simulink model "wrist_imu_main"  (R2025a)
settings: Solver=FixedStepDiscrete  StartTime=0.0  StopTime=T  FixedStep=Ts  RelTol=1e-3
undefined symbols (not defined in the file): imu
settings Model: Creator=CSY  LastModifiedBy=CSY

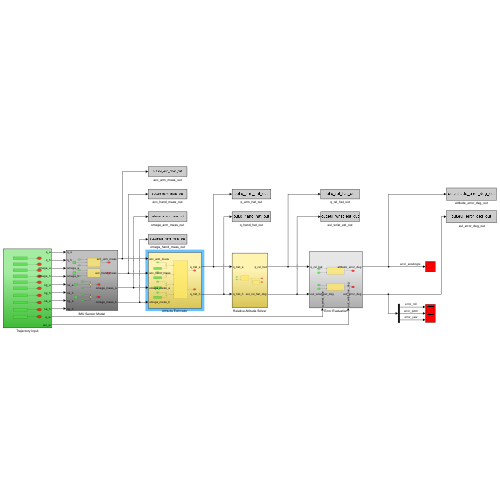
[thumbnail: Simulink's stored preview of the top-level diagram]
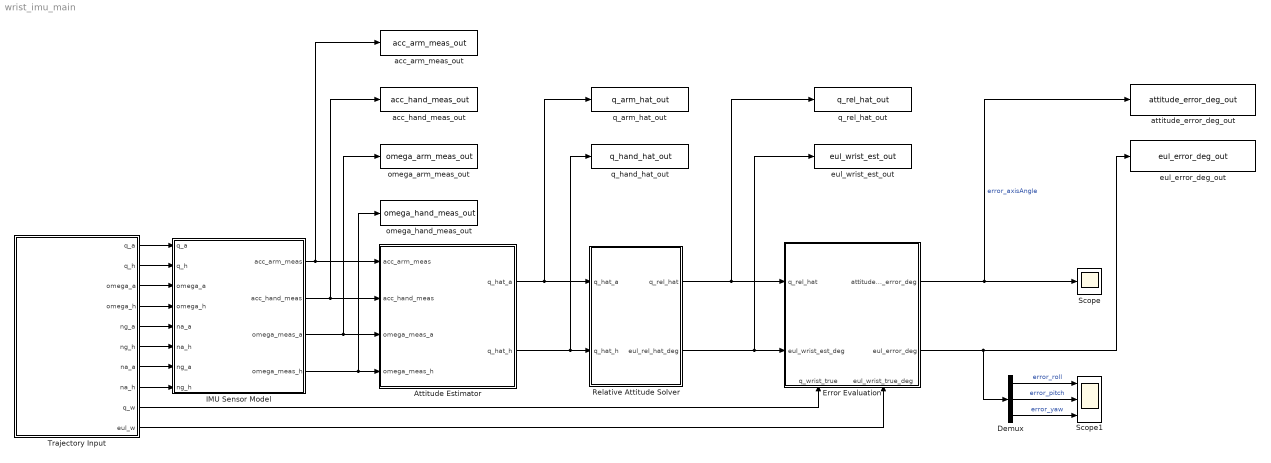
== system wrist_imu_main ==
  " eul_error_deg_out" : ToWorkspace  VariableName=eul_error_deg_out  SaveFormat=Timeseries  SampleTime=-1
  Attitude Estimator : Subsystem
  Demux : Demux  Outputs=3
  Error Evaluation : Subsystem
      settings: PortSchema="{\"entries\":[{\"content\":{\"sides\":[{\"content\":{\"connectorIds\":[\"In1\",\"In2\"]},\"type\":\"ConnectorPlacement.EquallySpacedRectSide\",\"uuid\":\"abe2ae72-a5a0-403c-9e03-1b4f6d4d0d67\"},{\"content\":{\"connectorIds\":[\"Out1\",\"Out2\"],\"side\":\"RIGHT\"},\"type\":\"ConnectorPlacement.EquallySpacedRectSide\",\"uuid\":\"685a4192-adf4-4593-bc2e-0bd30f7cac66\"},{\"content\":{\"side\":\"TOP\"},\"type\":\"ConnectorPlacement.EquallySpacedRectSide\",\"uuid\":\"39d5cefb-5657-4ba3-9dd7-93d12642c754\"},{\"content\":{\"connectorIds\":[\"In3\",\"In4\"],\"side\":\"BOTTOM\"},\"type\":\"ConnectorPlacement.EquallySpacedRectSide\",\"uuid\":\"5c41fd23-46de-49da-8620-9a3bda566928\"}]},\"type\":\"ConnectorPlacement.EquallySpacedConnector\",\"uuid\":\"e8722cc7-0898-4a9c-a259-ee97117e6560\"}],\"packageUris\":[\"http://schema.mathworks.com/mf0/Connector/R2020b\"],\"version\":\"1.0\"}"
  IMU Sensor Model : Subsystem
  Relative Attitude Solver : Subsystem
  Scope : Scope
      settings: ActiveDisplayYMinimum=-0.17689613299070039  ActiveDisplayYMaximum=0.60715026770063385
  Scope1 : Scope  NumInputPorts=3
      settings: ActiveDisplayYMinimum=-51.230869792156561  ActiveDisplayYMaximum=63.683087774127145
  Trajectory Input : Subsystem
  acc_arm_meas_out : ToWorkspace  VariableName=acc_arm_meas_out  SaveFormat=Timeseries  SampleTime=-1
  acc_hand_meas_out : ToWorkspace  VariableName=acc_hand_meas_out  SaveFormat=Timeseries  SampleTime=-1
  attitude_error_deg_out : ToWorkspace  VariableName=attitude_error_deg_out  SaveFormat=Timeseries  SampleTime=-1
  eul_wrist_est_out : ToWorkspace  VariableName=eul_wrist_est_out  SaveFormat=Timeseries  SampleTime=-1
  omega_arm_meas_out : ToWorkspace  VariableName=omega_arm_meas_out  SaveFormat=Timeseries  SampleTime=-1
  omega_hand_meas_out : ToWorkspace  VariableName=omega_hand_meas_out  SaveFormat=Timeseries  SampleTime=-1
  q_arm_hat_out : ToWorkspace  VariableName=q_arm_hat_out  SaveFormat=Timeseries  SampleTime=-1
  q_hand_hat_out : ToWorkspace  VariableName=q_hand_hat_out  SaveFormat=Timeseries  SampleTime=-1
  q_rel_hat_out : ToWorkspace  VariableName=q_rel_hat_out  SaveFormat=Timeseries  SampleTime=-1
  wires:
  Trajectory Input/3(omega_a) -> IMU Sensor Model/3(omega_a)
  Trajectory Input/4(omega_h) -> IMU Sensor Model/4(omega_h)
  IMU Sensor Model/3(omega_meas_a) -> omega_arm_meas_out/1, Attitude Estimator/3(omega_meas_a)
  IMU Sensor Model/4(omega_meas_h) -> omega_hand_meas_out/1, Attitude Estimator/4(omega_meas_h)
  Attitude Estimator/1(q_hat_a) -> Relative Attitude Solver/1(q_hat_a), q_arm_hat_out/1
  Attitude Estimator/2(q_hat_h) -> q_hand_hat_out/1, Relative Attitude Solver/2(q_hat_h)
  Relative Attitude Solver/1(q_rel_hat) -> q_rel_hat_out/1, Error Evaluation/1(q_rel_hat)
  Relative Attitude Solver/2(eul_rel_hat_deg) -> eul_wrist_est_out/1, Error Evaluation/2(eul_wrist_est_deg)
  Trajectory Input/9(q_w) -> Error Evaluation/3(q_wrist_true)
  Trajectory Input/10(eul_w) -> Error Evaluation/4(eul_wrist_true_deg)
  Error Evaluation/1(attitude_error_deg) -> attitude_error_deg_out/1, Scope/1  "error_axisAngle"
  Error Evaluation/2(eul_error_deg) -> Demux/1, " eul_error_deg_out"/1
  Demux/2 -> Scope1/2  "error_pitch"
  Demux/1 -> Scope1/1  "error_roll"
  Demux/3 -> Scope1/3  "error_yaw"
  Trajectory Input/1(q_a) -> IMU Sensor Model/1(q_a)
  Trajectory Input/2(q_h) -> IMU Sensor Model/2(q_h)
  IMU Sensor Model/1(acc_arm_meas) -> acc_arm_meas_out/1, Attitude Estimator/1(acc_arm_meas)
  IMU Sensor Model/2(acc_hand_meas) -> acc_hand_meas_out/1, Attitude Estimator/2(acc_hand_meas)
  Trajectory Input/5(ng_a) -> IMU Sensor Model/5(na_a)
  Trajectory Input/6(ng_h) -> IMU Sensor Model/6(na_h)
  Trajectory Input/7(na_a) -> IMU Sensor Model/7(ng_a)
  Trajectory Input/8(na_h) -> IMU Sensor Model/8(ng_h)

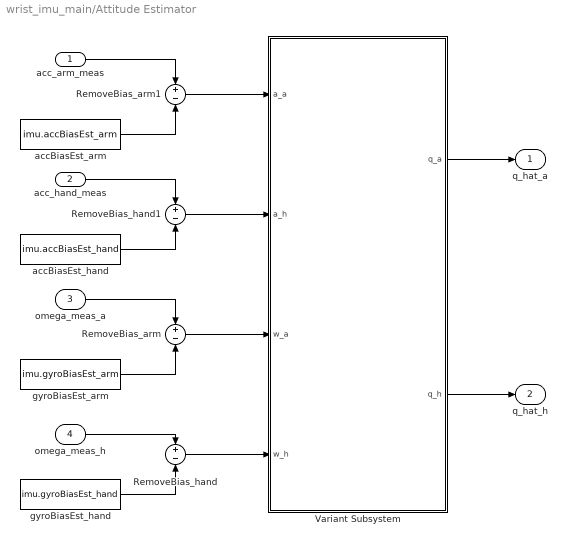
== system wrist_imu_main/Attitude Estimator ==
  acc_arm_meas : Inport
  acc_hand_meas : Inport  Port=2
  omega_meas_a : Inport  Port=3
  omega_meas_h : Inport  Port=4
  RemoveBias_arm : Sum  Inputs=+-
  RemoveBias_arm1 : Sum  Inputs=+-
  RemoveBias_hand : Sum  Inputs=+-
  RemoveBias_hand1 : Sum  Inputs=+-
  Variant Subsystem : Subsystem  Variant=on
  accBiasEst_arm : Constant  Value=imu.accBiasEst_arm
  accBiasEst_hand : Constant  Value=imu.accBiasEst_hand
  gyroBiasEst_arm : Constant  Value=imu.gyroBiasEst_arm
  gyroBiasEst_hand : Constant  Value=imu.gyroBiasEst_hand
  q_hat_a : Outport
  q_hat_h : Outport  Port=2
  wires:
  omega_meas_a/1 -> RemoveBias_arm/1
  gyroBiasEst_arm/1 -> RemoveBias_arm/2
  omega_meas_h/1 -> RemoveBias_hand/1
  gyroBiasEst_hand/1 -> RemoveBias_hand/2
  RemoveBias_arm/1 -> Variant Subsystem/3(w_a)
  Variant Subsystem/1(q_a) -> q_hat_a/1
  RemoveBias_hand/1 -> Variant Subsystem/4(w_h)
  Variant Subsystem/2(q_h) -> q_hat_h/1
  acc_arm_meas/1 -> RemoveBias_arm1/1
  acc_hand_meas/1 -> RemoveBias_hand1/1
  accBiasEst_arm/1 -> RemoveBias_arm1/2
  RemoveBias_arm1/1 -> Variant Subsystem/1(a_a)
  accBiasEst_hand/1 -> RemoveBias_hand1/2
  RemoveBias_hand1/1 -> Variant Subsystem/2(a_h)

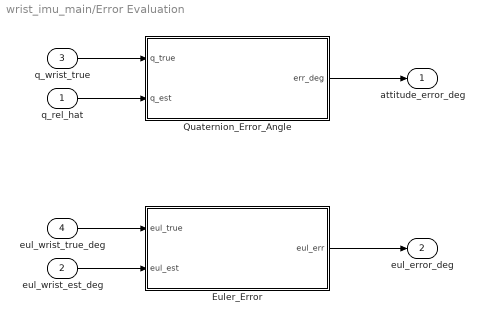
== system wrist_imu_main/Error Evaluation ==
  q_rel_hat : Inport
  eul_wrist_est_deg : Inport  Port=2
  q_wrist_true : Inport  Port=3
  eul_wrist_true_deg : Inport  Port=4
  Euler_Error : MATLAB Function  TreatAsAtomicUnit=on
  Quaternion_Error_Angle : MATLAB Function  TreatAsAtomicUnit=on
  attitude_error_deg : Outport
  eul_error_deg : Outport  Port=2
  wires:
  q_wrist_true/1 -> Quaternion_Error_Angle/1(q_true)
  q_rel_hat/1 -> Quaternion_Error_Angle/2(q_est)
  Quaternion_Error_Angle/1(err_deg) -> attitude_error_deg/1
  eul_wrist_true_deg/1 -> Euler_Error/1(eul_true)
  eul_wrist_est_deg/1 -> Euler_Error/2(eul_est)
  Euler_Error/1(eul_err) -> eul_error_deg/1

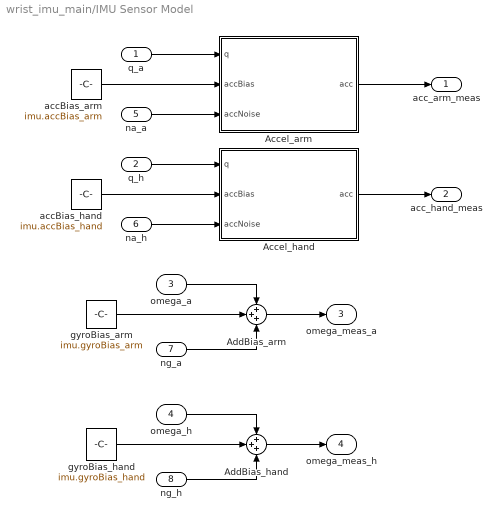
== system wrist_imu_main/IMU Sensor Model ==
  q_a : Inport
  q_h : Inport  Port=2
  omega_a : Inport  Port=3
  omega_h : Inport  Port=4
  na_a : Inport  Port=5
  na_h : Inport  Port=6
  ng_a : Inport  Port=7
  ng_h : Inport  Port=8
  Accel_arm : MATLAB Function  TreatAsAtomicUnit=on
  Accel_hand : MATLAB Function  TreatAsAtomicUnit=on
  AddBias_arm : Sum  Inputs=+++
  AddBias_hand : Sum  Inputs=+++
  accBias_arm : Constant  Value=imu.accBias_arm
  accBias_hand : Constant  Value=imu.accBias_hand
  gyroBias_arm : Constant  Value=imu.gyroBias_arm
  gyroBias_hand : Constant  Value=imu.gyroBias_hand
  acc_arm_meas : Outport
  acc_hand_meas : Outport  Port=2
  omega_meas_a : Outport  Port=3
  omega_meas_h : Outport  Port=4
  wires:
  omega_a/1 -> AddBias_arm/1
  gyroBias_arm/1 -> AddBias_arm/2
  AddBias_arm/1 -> omega_meas_a/1
  omega_h/1 -> AddBias_hand/1
  gyroBias_hand/1 -> AddBias_hand/2
  AddBias_hand/1 -> omega_meas_h/1
  q_h/1 -> Accel_hand/1(q)
  q_a/1 -> Accel_arm/1(q)
  Accel_arm/1(acc) -> acc_arm_meas/1
  Accel_hand/1(acc) -> acc_hand_meas/1
  accBias_hand/1 -> Accel_hand/2(accBias)
  accBias_arm/1 -> Accel_arm/2(accBias)
  na_h/1 -> Accel_hand/3(accNoise)
  na_a/1 -> Accel_arm/3(accNoise)
  ng_h/1 -> AddBias_hand/3
  ng_a/1 -> AddBias_arm/3

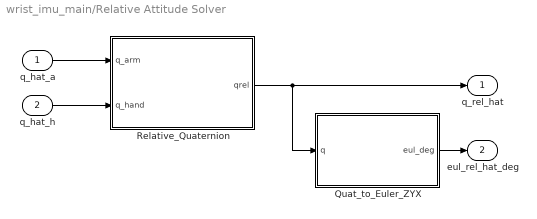
== system wrist_imu_main/Relative Attitude Solver ==
  q_hat_a : Inport
  q_hat_h : Inport  Port=2
  Quat_to_Euler_ZYX : MATLAB Function  TreatAsAtomicUnit=on
  Relative_Quaternion : MATLAB Function  TreatAsAtomicUnit=on
  q_rel_hat : Outport
  eul_rel_hat_deg : Outport  Port=2
  wires:
  q_hat_a/1 -> Relative_Quaternion/1(q_arm)
  q_hat_h/1 -> Relative_Quaternion/2(q_hand)
  Relative_Quaternion/1(qrel) -> Quat_to_Euler_ZYX/1(q), q_rel_hat/1
  Quat_to_Euler_ZYX/1(eul_deg) -> eul_rel_hat_deg/1

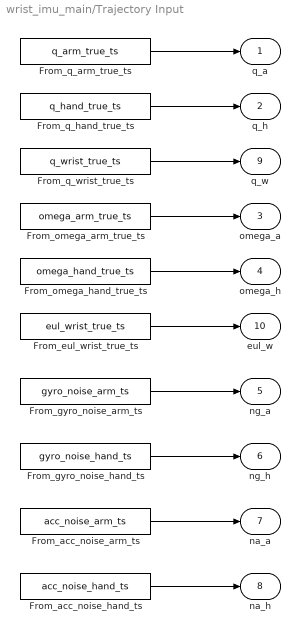
== system wrist_imu_main/Trajectory Input ==
  From_acc_noise_arm_ts : FromWorkspace  VariableName=acc_noise_arm_ts
  From_acc_noise_hand_ts : FromWorkspace  VariableName=acc_noise_hand_ts
  From_eul_wrist_true_ts : FromWorkspace  VariableName=eul_wrist_true_ts
  From_gyro_noise_arm_ts : FromWorkspace  VariableName=gyro_noise_arm_ts
  From_gyro_noise_hand_ts : FromWorkspace  VariableName=gyro_noise_hand_ts
  From_omega_arm_true_ts : FromWorkspace  VariableName=omega_arm_true_ts
  From_omega_hand_true_ts : FromWorkspace  VariableName=omega_hand_true_ts
  From_q_arm_true_ts : FromWorkspace  VariableName=q_arm_true_ts
  From_q_hand_true_ts : FromWorkspace  VariableName=q_hand_true_ts
  From_q_wrist_true_ts : FromWorkspace  VariableName=q_wrist_true_ts
  q_a : Outport
  q_h : Outport  Port=2
  omega_a : Outport  Port=3
  omega_h : Outport  Port=4
  ng_a : Outport  Port=5
  ng_h : Outport  Port=6
  na_a : Outport  Port=7
  na_h : Outport  Port=8
  q_w : Outport  Port=9
  eul_w : Outport  Port=10
  wires:
  From_q_arm_true_ts/1 -> q_a/1
  From_q_hand_true_ts/1 -> q_h/1
  From_q_wrist_true_ts/1 -> q_w/1
  From_omega_arm_true_ts/1 -> omega_a/1
  From_omega_hand_true_ts/1 -> omega_h/1
  From_eul_wrist_true_ts/1 -> eul_w/1
  From_gyro_noise_arm_ts/1 -> ng_a/1
  From_gyro_noise_hand_ts/1 -> ng_h/1
  From_acc_noise_arm_ts/1 -> na_a/1
  From_acc_noise_hand_ts/1 -> na_h/1

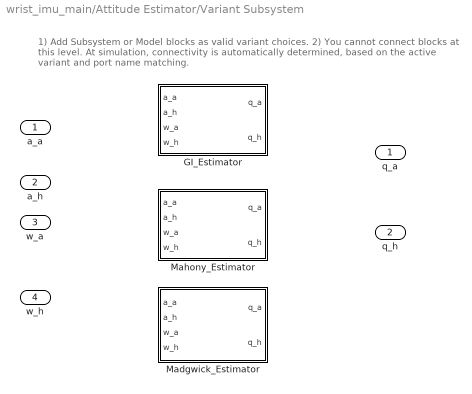
== system wrist_imu_main/Attitude Estimator/Variant Subsystem ==
  note: 1) Add Subsystem or Model blocks as valid variant choices.
      | 2) You cannot connect blocks at this level. At simulation, connectivity is automatically
      | determined, based on the active variant and port name matching.
  a_a : Inport
  a_h : Inport  Port=2
  w_a : Inport  Port=3
  w_h : Inport  Port=4
  GI_Estimator : Subsystem  VariantControl=ESTIMATOR == 1
  Madgwick_Estimator : Subsystem  VariantControl=ESTIMATOR == 3
  Mahony_Estimator : Subsystem  VariantControl=ESTIMATOR == 2
  q_a : Outport
  q_h : Outport  Port=2

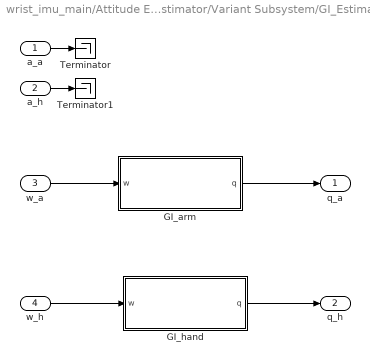
== system wrist_imu_main/Attitude Estimator/Variant Subsystem/GI_Estimator ==
  a_a : Inport
  a_h : Inport  Port=2
  w_a : Inport  Port=3
  w_h : Inport  Port=4
  GI_arm : MATLAB Function  TreatAsAtomicUnit=on
  GI_hand : MATLAB Function  TreatAsAtomicUnit=on
  Terminator : Terminator
  Terminator1 : Terminator
  q_a : Outport
  q_h : Outport  Port=2
  wires:
  w_h/1 -> GI_hand/1(w)
  GI_arm/1(q) -> q_a/1
  GI_hand/1(q) -> q_h/1
  w_a/1 -> GI_arm/1(w)
  a_a/1 -> Terminator/1
  a_h/1 -> Terminator1/1

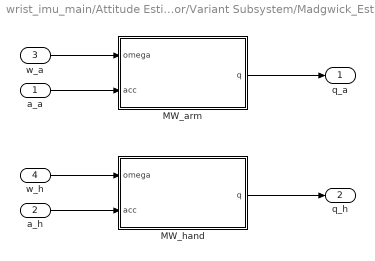
== system wrist_imu_main/Attitude Estimator/Variant Subsystem/Madgwick_Estimator ==
  a_a : Inport
  a_h : Inport  Port=2
  w_a : Inport  Port=3
  w_h : Inport  Port=4
  MW_arm : MATLAB Function  TreatAsAtomicUnit=on
  MW_hand : MATLAB Function  TreatAsAtomicUnit=on
  q_a : Outport
  q_h : Outport  Port=2
  wires:
  w_h/1 -> MW_hand/1(omega)
  w_a/1 -> MW_arm/1(omega)
  MW_hand/1(q) -> q_h/1
  MW_arm/1(q) -> q_a/1
  a_a/1 -> MW_arm/2(acc)
  a_h/1 -> MW_hand/2(acc)

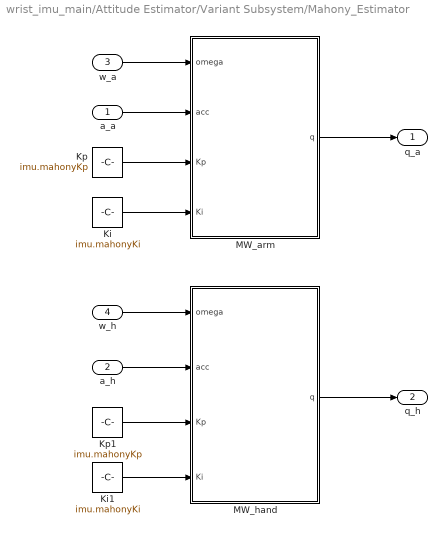
== system wrist_imu_main/Attitude Estimator/Variant Subsystem/Mahony_Estimator ==
  a_a : Inport
  a_h : Inport  Port=2
  w_a : Inport  Port=3
  w_h : Inport  Port=4
  Ki : Constant  Value=imu.mahonyKi
  Ki1 : Constant  Value=imu.mahonyKi
  Kp : Constant  Value=imu.mahonyKp
  Kp1 : Constant  Value=imu.mahonyKp
  MW_arm : MATLAB Function  TreatAsAtomicUnit=on
  MW_hand : MATLAB Function  TreatAsAtomicUnit=on
  q_a : Outport
  q_h : Outport  Port=2
  wires:
  w_a/1 -> MW_arm/1(omega)
  w_h/1 -> MW_hand/1(omega)
  MW_arm/1(q) -> q_a/1
  a_h/1 -> MW_hand/2(acc)
  MW_hand/1(q) -> q_h/1
  a_a/1 -> MW_arm/2(acc)
  Kp/1 -> MW_arm/3(Kp)
  Ki/1 -> MW_arm/4(Ki)
  Kp1/1 -> MW_hand/3(Kp)
  Ki1/1 -> MW_hand/4(Ki)

== matlab function wrist_imu_main/IMU Sensor Model/Accel_hand ==
  data: q input; acc output; accBias input; accNoise input
function acc = Accel_Model(q, accBias, accNoise)
%#codegen
% q: [w x y z], body -> world
% acc: body frame accelerometer output, m/s^2

q = q(:);
q = q / norm(q);

w = q(1);
x = q(2);
y = q(3);
z = q(4);

R = zeros(3,3);

R(1,1) = 1 - 2*(y^2 + z^2);
R(1,2) = 2*(x*y - w*z);
R(1,3) = 2*(x*z + w*y);

R(2,1) = 2*(x*y + w*z);
R(2,2) = 1 - 2*(x^2 + z^2);
R(2,3) = 2*(y*z - w*x);

R(3,1) = 2*(x*z - w*y);
R(3,2) = 2*(y*z + w*x);
R(3,3) = 1 - 2*(x^2 + y^2);

g_W = [0; 0; 9.81];

acc = R' * g_W + accBias(:) + accNoise(:);
end

== matlab function wrist_imu_main/IMU Sensor Model/Accel_arm ==
  data: q input; acc output; accBias input; accNoise input
function acc = Accel_Model(q, accBias, accNoise)
%#codegen
% q: [w x y z], body -> world
% acc: body frame accelerometer output, m/s^2

q = q(:);
q = q / norm(q);

w = q(1);
x = q(2);
y = q(3);
z = q(4);

R = zeros(3,3);

R(1,1) = 1 - 2*(y^2 + z^2);
R(1,2) = 2*(x*y - w*z);
R(1,3) = 2*(x*z + w*y);

R(2,1) = 2*(x*y + w*z);
R(2,2) = 1 - 2*(x^2 + z^2);
R(2,3) = 2*(y*z - w*x);

R(3,1) = 2*(x*z - w*y);
R(3,2) = 2*(y*z + w*x);
R(3,3) = 1 - 2*(x^2 + y^2);

g_W = [0; 0; 9.81];

acc = R' * g_W + accBias(:) + accNoise(:);
end

== matlab function wrist_imu_main/Relative Attitude Solver/Relative_Quaternion ==
  data: q_arm input; qrel output; q_hand input
function qrel = Relative_Quaternion(q_arm, q_hand)
%#codegen
% qrel = q_arm^{-1} ⊗ q_hand
% 四元数格式：[w x y z]，标量在前

q_arm = q_arm(:);
q_hand = q_hand(:);

q_arm = q_arm / norm(q_arm);
q_hand = q_hand / norm(q_hand);

% q_arm 的逆：单位四元数的逆等于共轭
q1 = zeros(4,1);
q1(1) = q_arm(1);
q1(2:4) = -q_arm(2:4);

q2 = q_hand;

% qrel = q1 ⊗ q2
s1 = q1(1);
v1 = q1(2:4);
s2 = q2(1);
v2 = q2(2:4);

qrel = zeros(4,1);
qrel(1) = s1*s2 - dot(v1,v2);
qrel(2:4) = s1*v2 + s2*v1 + cross(v1,v2);

qrel = qrel / norm(qrel);

% 统一符号，避免 q 和 -q 跳变
if qrel(1) < 0
    qrel = -qrel;
end
end

== matlab function wrist_imu_main/Relative Attitude Solver/Quat_to_Euler_ZYX ==
  data: q input; eul_deg output
function eul_deg = Quat_to_Euler_ZYX(q)
%#codegen
% 输入 q: [w x y z]
% 输出 eul_deg = [roll pitch yaw]，单位 deg
% 欧拉角顺序：ZYX，即 R = Rz(yaw) * Ry(pitch) * Rx(roll)

q = q(:);
q = q / norm(q);

w = q(1);
x = q(2);
y = q(3);
z = q(4);

R11 = 1 - 2*(y^2 + z^2);
R21 = 2*(x*y + w*z);
R31 = 2*(x*z - w*y);
R32 = 2*(y*z + w*x);
R33 = 1 - 2*(x^2 + y^2);

% 防止数值误差导致 asin 输入略超 [-1,1]
v = -R31;
if v > 1
    v = 1;
elseif v < -1
    v = -1;
end

pitch = asin(v);
roll  = atan2(R32, R33);
yaw   = atan2(R21, R11);

eul_deg = [roll; pitch; yaw] * 180/pi;

== matlab function wrist_imu_main/Error Evaluation/Quaternion_Error_Angle ==
  data: q_true input; err_deg output; q_est input
function err_deg = Quaternion_Error_Angle(q_true, q_est)
%#codegen
% 计算 q_true 和 q_est 之间的姿态误差角，单位 deg

q_true = q_true(:);
q_est = q_est(:);

q_true = q_true / norm(q_true);
q_est = q_est / norm(q_est);

% qerr = q_true^{-1} ⊗ q_est
q1 = zeros(4,1);
q1(1) = q_true(1);
q1(2:4) = -q_true(2:4);

q2 = q_est;

s1 = q1(1);
v1 = q1(2:4);
s2 = q2(1);
v2 = q2(2:4);

qerr = zeros(4,1);
qerr(1) = s1*s2 - dot(v1,v2);
qerr(2:4) = s1*v2 + s2*v1 + cross(v1,v2);
qerr = qerr / norm(qerr);

% q 和 -q 表示同一姿态，所以取 abs
c = abs(qerr(1));
if c > 1
    c = 1;
end

err_deg = 2 * acos(c) * 180/pi;
end

== matlab function wrist_imu_main/Error Evaluation/Euler_Error ==
  data: eul_true input; eul_err output; eul_est input
function eul_err = Euler_Error(eul_true, eul_est)
%#codegen
% 输入单位 deg，输出 eul_est - eul_true

eul_true = eul_true(:);
eul_est = eul_est(:);

eul_err = zeros(3,1);
eul_err = eul_est - eul_true;

% 简单处理角度跨越 ±180 的情况
for i = 1:3
    if eul_err(i) > 180
        eul_err(i) = eul_err(i) - 360;
    elseif eul_err(i) < -180
        eul_err(i) = eul_err(i) + 360;
    end
end
end

== matlab function wrist_imu_main/Attitude Estimator/Variant Subsystem/GI_Estimator/GI_arm ==
  data: w input; q output
function q = GI_Quat_Integrator(w)
%#codegen

% 输入 w: 3维角速度，单位 rad/s
% 输出 q: 4x1 四元数 [w x y z]

persistent qk
Ts = 0.01;

if isempty(qk)
    qk = zeros(4,1);
    qk(1) = 1;
end

w = w(:);
theta = norm(w) * Ts;

if theta < 1e-12
    dq = zeros(4,1);
    dq(1) = 1;
    dq(2:4) = 0.5 * w * Ts;
else
    axis = w / norm(w);
    dq = zeros(4,1);
    dq(1) = cos(theta/2);
    dq(2:4) = axis * sin(theta/2);
end

% qk = qk ⊗ dq
s1 = qk(1);
v1 = qk(2:4);
s2 = dq(1);
v2 = dq(2:4);

qnew = zeros(4,1);
qnew(1) = s1*s2 - dot(v1,v2);
qnew(2:4) = s1*v2 + s2*v1 + cross(v1,v2);

qk = qnew / norm(qnew);
q = qk;
end

== matlab function wrist_imu_main/Attitude Estimator/Variant Subsystem/GI_Estimator/GI_hand ==
  data: w input; q output
function q = GI_Quat_Integrator(w)
%#codegen

% 输入 w: 3维角速度，单位 rad/s
% 输出 q: 4x1 四元数 [w x y z]

persistent qk
Ts = 0.01;

if isempty(qk)
    qk = zeros(4,1);
    qk(1) = 1;
end

w = w(:);
theta = norm(w) * Ts;

if theta < 1e-12
    dq = zeros(4,1);
    dq(1) = 1;
    dq(2:4) = 0.5 * w * Ts;
else
    axis = w / norm(w);
    dq = zeros(4,1);
    dq(1) = cos(theta/2);
    dq(2:4) = axis * sin(theta/2);
end

% qk = qk ⊗ dq
s1 = qk(1);
v1 = qk(2:4);
s2 = dq(1);
v2 = dq(2:4);

qnew = zeros(4,1);
qnew(1) = s1*s2 - dot(v1,v2);
qnew(2:4) = s1*v2 + s2*v1 + cross(v1,v2);

qk = qnew / norm(qnew);
q = qk;
end

== matlab function wrist_imu_main/Attitude Estimator/Variant Subsystem/Madgwick_Estimator/MW_arm ==
  data: omega input; q output; acc input
function q = Mahony_IMU(omega, acc)
%#codegen
% omega: 3x1 rad/s
% acc:   3x1 m/s^2
% q:     4x1 quaternion [w x y z]
%
% q 表示 body -> world 的姿态

persistent qk intErr

Ts = 0.01;
Kp = 2.0;
Ki = 0.05;

if isempty(qk)
    qk = [1;0;0;0];
    intErr = [0;0;0];
end

omega = omega(:);
acc = acc(:);

% 加速度归一化，只保留方向
accNorm = norm(acc);
if accNorm > 1e-8
    a = acc / accNorm;
else
    a = [0;0;1];
end

% 当前四元数
qk = qk / norm(qk);

w = qk(1);
x = qk(2);
y = qk(3);
z = qk(4);

% R: body -> world
R = zeros(3,3);
R(1,1) = 1 - 2*(y^2 + z^2);
R(1,2) = 2*(x*y - w*z);
R(1,3) = 2*(x*z + w*y);

R(2,1) = 2*(x*y + w*z);
R(2,2) = 1 - 2*(x^2 + z^2);
R(2,3) = 2*(y*z - w*x);

R(3,1) = 2*(x*z - w*y);
R(3,2) = 2*(y*z + w*x);
R(3,3) = 1 - 2*(x^2 + y^2);

% 预测的重力方向在 body 坐标系下的表达
g_world = [0;0;1];
g_hat_body = R' * g_world;

% 姿态误差：测得重力方向 vs 预测重力方向
e = cross(a, g_hat_body);

% 积分项，用于补偿陀螺零偏
intErr = intErr + e * Ts;

% 修正角速度
omega_corr = omega + Kp * e + Ki * intErr;

% 四元数积分
theta = norm(omega_corr) * Ts;

if theta < 1e-12
    dq = [1; 0.5 * omega_corr * Ts];
else
    axis = omega_corr / norm(omega_corr);
    dq = [cos(theta/2); axis * sin(theta/2)];
end

% qk = qk ⊗ dq
s1 = qk(1); v1 = qk(2:4);
s2 = dq(1); v2 = dq(2:4);

qnew = zeros(4,1);
qnew(1) = s1*s2 - dot(v1,v2);
qnew(2:4) = s1*v2 + s2*v1 + cross(v1,v2);

qk = qnew / norm(qnew);
q = qk;
end

== matlab function wrist_imu_main/Attitude Estimator/Variant Subsystem/Madgwick_Estimator/MW_hand ==
  data: omega input; q output; acc input
function q = Mahony_IMU(omega, acc)
%#codegen
% omega: 3x1 rad/s
% acc:   3x1 m/s^2
% q:     4x1 quaternion [w x y z]
%
% q 表示 body -> world 的姿态

persistent qk intErr

Ts = 0.01;
Kp = 2.0;
Ki = 0.05;

if isempty(qk)
    qk = [1;0;0;0];
    intErr = [0;0;0];
end

omega = omega(:);
acc = acc(:);

% 加速度归一化，只保留方向
accNorm = norm(acc);
if accNorm > 1e-8
    a = acc / accNorm;
else
    a = [0;0;1];
end

% 当前四元数
qk = qk / norm(qk);

w = qk(1);
x = qk(2);
y = qk(3);
z = qk(4);

% R: body -> world
R = zeros(3,3);
R(1,1) = 1 - 2*(y^2 + z^2);
R(1,2) = 2*(x*y - w*z);
R(1,3) = 2*(x*z + w*y);

R(2,1) = 2*(x*y + w*z);
R(2,2) = 1 - 2*(x^2 + z^2);
R(2,3) = 2*(y*z - w*x);

R(3,1) = 2*(x*z - w*y);
R(3,2) = 2*(y*z + w*x);
R(3,3) = 1 - 2*(x^2 + y^2);

% 预测的重力方向在 body 坐标系下的表达
g_world = [0;0;1];
g_hat_body = R' * g_world;

% 姿态误差：测得重力方向 vs 预测重力方向
e = cross(a, g_hat_body);

% 积分项，用于补偿陀螺零偏
intErr = intErr + e * Ts;

% 修正角速度
omega_corr = omega + Kp * e + Ki * intErr;

% 四元数积分
theta = norm(omega_corr) * Ts;

if theta < 1e-12
    dq = [1; 0.5 * omega_corr * Ts];
else
    axis = omega_corr / norm(omega_corr);
    dq = [cos(theta/2); axis * sin(theta/2)];
end

% qk = qk ⊗ dq
s1 = qk(1); v1 = qk(2:4);
s2 = dq(1); v2 = dq(2:4);

qnew = zeros(4,1);
qnew(1) = s1*s2 - dot(v1,v2);
qnew(2:4) = s1*v2 + s2*v1 + cross(v1,v2);

qk = qnew / norm(qnew);
q = qk;
end

== matlab function wrist_imu_main/Attitude Estimator/Variant Subsystem/Mahony_Estimator/MW_arm ==
  data: omega input; q output; acc input; Kp input; Ki input
function q = Mahony_IMU(omega, acc, Kp, Ki)
%#codegen
% omega: 3x1 rad/s
% acc:   3x1 m/s^2
% q:     4x1 quaternion [w x y z]
%
% q 表示 body -> world 的姿态

persistent qk intErr

Ts = 0.01;

if isempty(qk)
    qk = [1;0;0;0];
    intErr = [0;0;0];
end

omega = omega(:);
acc = acc(:);

% 加速度归一化，只保留方向
accNorm = norm(acc);
if accNorm > 1e-8
    a = acc / accNorm;
else
    a = [0;0;1];
end

% 当前四元数
qk = qk / norm(qk);

w = qk(1);
x = qk(2);
y = qk(3);
z = qk(4);

% R: body -> world
R = zeros(3,3);
R(1,1) = 1 - 2*(y^2 + z^2);
R(1,2) = 2*(x*y - w*z);
R(1,3) = 2*(x*z + w*y);

R(2,1) = 2*(x*y + w*z);
R(2,2) = 1 - 2*(x^2 + z^2);
R(2,3) = 2*(y*z - w*x);

R(3,1) = 2*(x*z - w*y);
R(3,2) = 2*(y*z + w*x);
R(3,3) = 1 - 2*(x^2 + y^2);

% 预测的重力方向在 body 坐标系下的表达
g_world = [0;0;1];
g_hat_body = R' * g_world;

% 姿态误差：测得重力方向 vs 预测重力方向
e = cross(a, g_hat_body);
% e = cross(g_hat_body, a);

% 积分项，用于补偿陀螺零偏
intErr = intErr + e * Ts;

% 修正角速度
omega_corr = omega + Kp * e + Ki * intErr;

% 四元数积分
theta = norm(omega_corr) * Ts;

if theta < 1e-12
    dq = [1; 0.5 * omega_corr * Ts];
else
    axis = omega_corr / norm(omega_corr);
    dq = [cos(theta/2); axis * sin(theta/2)];
end

% qk = qk ⊗ dq
s1 = qk(1); v1 = qk(2:4);
s2 = dq(1); v2 = dq(2:4);

qnew = zeros(4,1);
qnew(1) = s1*s2 - dot(v1,v2);
qnew(2:4) = s1*v2 + s2*v1 + cross(v1,v2);

qk = qnew / norm(qnew);
q = qk;
end

== matlab function wrist_imu_main/Attitude Estimator/Variant Subsystem/Mahony_Estimator/MW_hand ==
  data: omega input; q output; acc input; Kp input; Ki input
function q = Mahony_IMU(omega, acc, Kp, Ki)
%#codegen
% omega: 3x1 rad/s
% acc:   3x1 m/s^2
% q:     4x1 quaternion [w x y z]
%
% q 表示 body -> world 的姿态

persistent qk intErr

Ts = 0.01;

if isempty(qk)
    qk = [1;0;0;0];
    intErr = [0;0;0];
end

omega = omega(:);
acc = acc(:);

% 加速度归一化，只保留方向
accNorm = norm(acc);
if accNorm > 1e-8
    a = acc / accNorm;
else
    a = [0;0;1];
end

% 当前四元数
qk = qk / norm(qk);

w = qk(1);
x = qk(2);
y = qk(3);
z = qk(4);

% R: body -> world
R = zeros(3,3);
R(1,1) = 1 - 2*(y^2 + z^2);
R(1,2) = 2*(x*y - w*z);
R(1,3) = 2*(x*z + w*y);

R(2,1) = 2*(x*y + w*z);
R(2,2) = 1 - 2*(x^2 + z^2);
R(2,3) = 2*(y*z - w*x);

R(3,1) = 2*(x*z - w*y);
R(3,2) = 2*(y*z + w*x);
R(3,3) = 1 - 2*(x^2 + y^2);

% 预测的重力方向在 body 坐标系下的表达
g_world = [0;0;1];
g_hat_body = R' * g_world;

% 姿态误差：测得重力方向 vs 预测重力方向
e = cross(a, g_hat_body);
% e = cross(g_hat_body, a);

% 积分项，用于补偿陀螺零偏
intErr = intErr + e * Ts;

% 修正角速度
omega_corr = omega + Kp * e + Ki * intErr;

% 四元数积分
theta = norm(omega_corr) * Ts;

if theta < 1e-12
    dq = [1; 0.5 * omega_corr * Ts];
else
    axis = omega_corr / norm(omega_corr);
    dq = [cos(theta/2); axis * sin(theta/2)];
end

% qk = qk ⊗ dq
s1 = qk(1); v1 = qk(2:4);
s2 = dq(1); v2 = dq(2:4);

qnew = zeros(4,1);
qnew(1) = s1*s2 - dot(v1,v2);
qnew(2:4) = s1*v2 + s2*v1 + cross(v1,v2);

qk = qnew / norm(qnew);
q = qk;
end
